simulink model "furuta_sim"  (R2020b)
settings: Solver=VariableStepAuto  StartTime=0.0  StopTime=10  MaxStep=1e-3  RelTol=1e-3
values from neighbouring files (symbols this model uses):
  A = A1    [furuta_script.m]    (also in practica2.m = [0 1; -2 -3])
  B = B1    [furuta_script.m]    (also in practica2.m = [10; 20])
  b1 = 1.00e-4    (= 0.0001)    [parameters.m]
  b2 = 2.80e-4    (= 0.00028)    [parameters.m]
  C = [1 0 0 0 0; 0 1 0 0 0]    [parameters.m]    (also in practica2.m = [1 0])
  CI = [-5*pi/180 -pi*5/180 0 0 0]    [furuta_script.m]
  g = 9.81    [parameters.m]
  J_hat_0 = J_hat_1+m2*L1^2    (= 0.0373463)    [parameters.m]
  J_hat_2 = J2+m2*l2^2    (= 0.0055028)    [parameters.m]
  K = acker(Pss.A, Pss.B, Pd)    [practica2_2.m]    (also in test_delete.m = Ka(1:3))
  Ki = -Ka(end)    [test_delete.m]
  Km = 0.090    (= 0.09)    [parameters.m]
  L = 0.005    [parameters.m]    (also in practica2_2.m = acker(Pss.A', Pss.c', Pdl)'; test_delete.m = acker(A',C',po)')
  L1 = 0.278    [parameters.m]
  l2 = 0.148    [parameters.m]
  m2 = 0.075    [parameters.m]
  n = length(A1)    [parameters.m]
  p = width(B1)    [parameters.m]    (also in test_delete.m = roots(conv([1 2*z*wn wn^2], [ 1 alpha*wn])))
  R = 7.80    (= 7.8)    [parameters.m]
undefined symbols (not defined in the file or in its folder): Kb, Nbar, Nbarb, Nbari
settings Model: Creator=jorgegonzales  LastModifiedBy=jorgegonzales

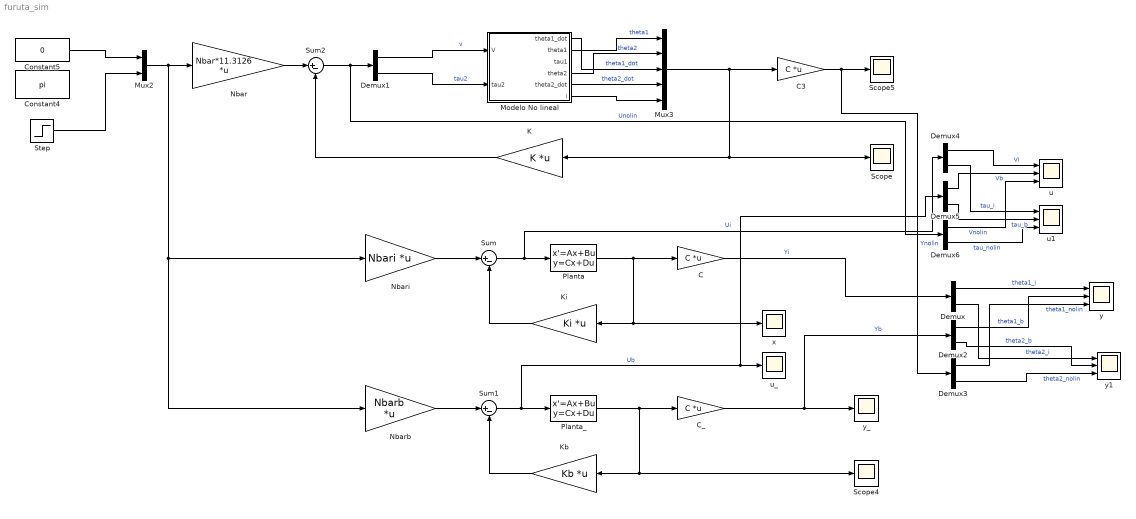
== system furuta_sim ==
  C : Gain  Gain=C  Multiplication=Matrix(K*u) (u vector)
  C3 : Gain  Gain=C  Multiplication=Matrix(K*u) (u vector)
  C_ : Gain  Gain=C  Multiplication=Matrix(K*u) (u vector)
  Constant4 : Constant  Value=pi
  Constant5 : Constant  Value=0
  Demux{,1..6} (7 alike) : Demux  Outputs=2
  K : Gain  Gain=K  Multiplication=Matrix(K*u) (u vector)
  Kb : Gain  Gain=Kb  Multiplication=Matrix(K*u) (u vector)
  Ki : Gain  Gain=Ki  Multiplication=Matrix(K*u) (u vector)
  Modelo No lineal : Subsystem
  Mux2 : Mux  Inputs=2
  Mux3 : Mux  Inputs=5
  Nbar : Gain  Gain=Nbar*11.3126  Multiplication=Matrix(K*u) (u vector)
  Nbarb : Gain  Gain=Nbarb  Multiplication=Matrix(K*u) (u vector)
  Nbari : Gain  Gain=Nbari  Multiplication=Matrix(K*u) (u vector)
  Planta : StateSpace  A=A  B=B  C=eye(n)  D=zeros(n,p)  InitialCondition=CI
  Planta_ : StateSpace  A=A  B=B  C=eye(n)  D=zeros(n,p)  InitialCondition=CI
  Scope : Scope
  Scope4 : Scope
  Scope5 : Scope
  Step : Step  Time=0.03  After=pi  SampleTime=0
  Sum : Sum  Inputs=|+-
  Sum1 : Sum  Inputs=|+-
  Sum2 : Sum  Inputs=|+-
  u : Scope  NumInputPorts=3
  u1 : Scope  NumInputPorts=3
  u_ : Scope
  x : Scope
  y : Scope  NumInputPorts=3
  y1 : Scope  NumInputPorts=3
  y_ : Scope
  wires:
  Ki/1 -> Sum/2
  Nbari/1 -> Sum/1
  Demux1/1 -> Modelo No lineal/1(V)  "v"
  Demux1/2 -> Modelo No lineal/2(tau2)  "tau2"
  C/1 -> Demux/1  "Yi"
  Planta/1 -> C/1, x/1, Ki/1
  Sum/1 -> Demux4/1, Planta/1  "Ui"
  Sum1/1 -> Demux5/1, u_/1, Planta_/1  "Ub"
  C_/1 -> Demux2/1, y_/1  "Yb"
  Planta_/1 -> Scope4/1, Kb/1, C_/1
  Nbarb/1 -> Sum1/1
  Kb/1 -> Sum1/2
  Constant5/1 -> Mux2/1
  Mux2/1 -> Nbarb/1, Nbari/1, Nbar/1
  Modelo No lineal/2(theta1) -> Mux3/1  "theta1"
  Modelo No lineal/4(theta2) -> Mux3/2  "theta2"
  Modelo No lineal/1(theta1_dot) -> Mux3/3  "theta1_dot"
  Modelo No lineal/5(theta2_dot) -> Mux3/4  "theta2_dot"
  Modelo No lineal/6(i) -> Mux3/5
  Mux3/1 -> C3/1, K/1, Scope/1
  C3/1 -> Demux3/1, Scope5/1  "Ynolin"
  Sum2/1 -> Demux6/1, Demux1/1  "Unolin"
  Nbar/1 -> Sum2/1
  K/1 -> Sum2/2
  Demux/1 -> y/1  "theta1_i"
  Demux2/1 -> y/2  "theta1_b"
  Demux3/1 -> y/3  "theta1_nolin"
  Demux/2 -> y1/1  "theta2_i"
  Demux2/2 -> y1/2  "theta2_b"
  Demux3/2 -> y1/3  "theta2_nolin"
  Demux4/1 -> u/1  "Vi"
  Demux4/2 -> u1/1  "tau_i"
  Demux5/1 -> u/2  "Vb"
  Demux5/2 -> u1/2  "tau_b"
  Demux6/1 -> u/3  "Vnolin"
  Demux6/2 -> u1/3  "tau_nolin"
  Step/1 -> Mux2/2

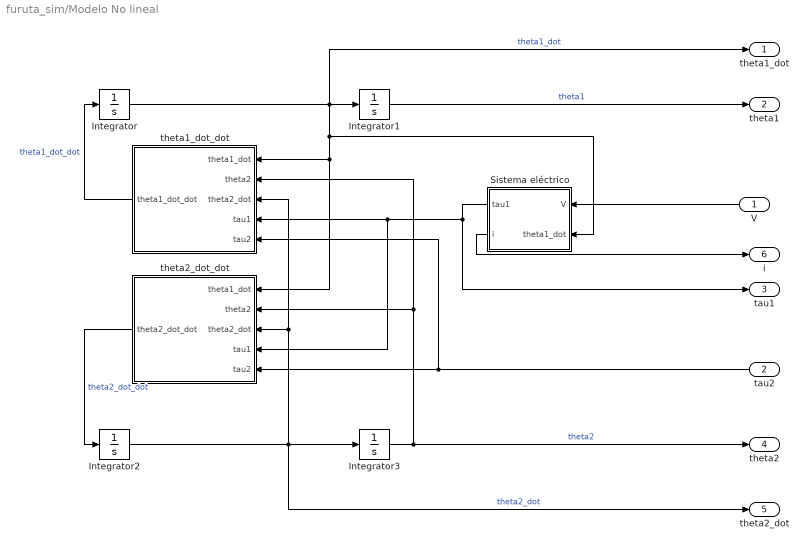
== system furuta_sim/Modelo No lineal ==
  V : Inport
  tau2 : Inport  Port=2
  Integrator : Integrator  InitialCondition=CI(3)
  Integrator1 : Integrator  InitialCondition=CI(1)
  Integrator2 : Integrator  InitialCondition=CI(4)
  Integrator3 : Integrator  InitialCondition=CI(2)
  Sistema eléctrico : Subsystem
  theta1_dot_dot : Subsystem
  theta2_dot_dot : Subsystem
  theta1_dot : Outport
  theta1 : Outport  Port=2
  tau1 : Outport  Port=3
  theta2 : Outport  Port=4
  theta2_dot : Outport  Port=5
  i : Outport  Port=6
  wires:
  Sistema eléctrico/1(tau1) -> tau1/1, theta2_dot_dot/4(tau1), theta1_dot_dot/4(tau1)
  theta1_dot_dot/1(theta1_dot_dot) -> Integrator/1  "theta1_dot_dot"
  V/1 -> Sistema eléctrico/1(V)
  Integrator3/1 -> theta2/1, theta2_dot_dot/2(theta2), theta1_dot_dot/2(theta2)  "theta2"
  tau2/1 -> theta1_dot_dot/5(tau2), theta2_dot_dot/5(tau2)
  theta2_dot_dot/1(theta2_dot_dot) -> Integrator2/1  "theta2_dot_dot"
  Integrator1/1 -> theta1/1  "theta1"
  Integrator2/1 -> theta2_dot/1, theta2_dot_dot/3(theta2_dot), theta1_dot_dot/3(theta2_dot), Integrator3/1  "theta2_dot"
  Integrator/1 -> theta1_dot/1, Sistema eléctrico/2(theta1_dot), theta1_dot_dot/1(theta1_dot), theta2_dot_dot/1(theta1_dot), Integrator1/1  "theta1_dot"
  Sistema eléctrico/2(i) -> i/1

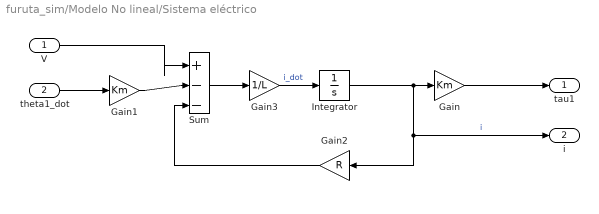
== system furuta_sim/Modelo No lineal/Sistema eléctrico ==
  V : Inport
  theta1_dot : Inport  Port=2
  Gain : Gain  Gain=Km
  Gain1 : Gain  Gain=Km
  Gain2 : Gain  Gain=R
  Gain3 : Gain  Gain=1/L
  Integrator : Integrator  InitialCondition=CI(5)
  Sum : Sum  Inputs=|+--
  tau1 : Outport
  i : Outport  Port=2
  wires:
  Integrator/1 -> i/1, Gain2/1, Gain/1  "i"
  Gain/1 -> tau1/1
  theta1_dot/1 -> Gain1/1
  Gain1/1 -> Sum/2
  V/1 -> Sum/1
  Gain2/1 -> Sum/3
  Gain3/1 -> Integrator/1  "i_dot"
  Sum/1 -> Gain3/1

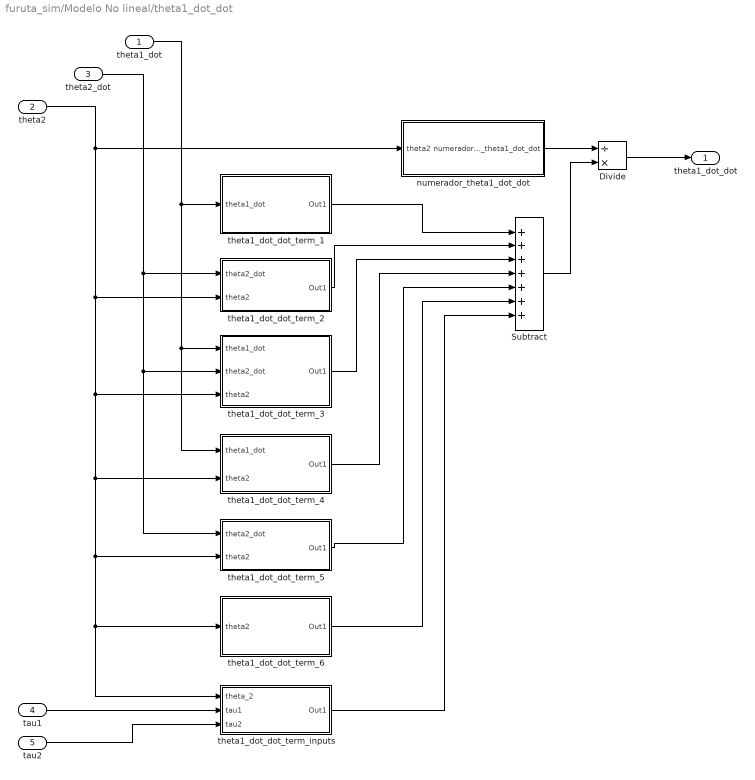
== system furuta_sim/Modelo No lineal/theta1_dot_dot ==
  theta1_dot : Inport
  theta2 : Inport  Port=2
  theta2_dot : Inport  Port=3
  tau1 : Inport  Port=4
  tau2 : Inport  Port=5
  Divide : Product  Inputs=/*
  Subtract : Sum  Inputs=+++++++
  numerador_theta1_dot_dot : Subsystem
  theta1_dot_dot_term_1 : Subsystem
  theta1_dot_dot_term_2 : Subsystem
  theta1_dot_dot_term_3 : Subsystem
  theta1_dot_dot_term_4 : Subsystem
  theta1_dot_dot_term_5 : Subsystem
  theta1_dot_dot_term_6 : Subsystem
  theta1_dot_dot_term_inputs : Subsystem
  theta1_dot_dot : Outport
  wires:
  theta1_dot_dot_term_4/1(Out1) -> Subtract/4
  theta1_dot/1 -> theta1_dot_dot_term_3/1(theta1_dot), theta1_dot_dot_term_4/1(theta1_dot), theta1_dot_dot_term_1/1(theta1_dot)
  theta1_dot_dot_term_3/1(Out1) -> Subtract/3
  theta1_dot_dot_term_5/1(Out1) -> Subtract/5
  theta1_dot_dot_term_2/1(Out1) -> Subtract/2
  theta1_dot_dot_term_1/1(Out1) -> Subtract/1
  theta2_dot/1 -> theta1_dot_dot_term_5/1(theta2_dot), theta1_dot_dot_term_3/2(theta2_dot), theta1_dot_dot_term_2/1(theta2_dot)
  theta2/1 -> numerador_theta1_dot_dot/1(theta2), theta1_dot_dot_term_4/2(theta2), theta1_dot_dot_term_6/1(theta2), theta1_dot_dot_term_inputs/1(theta_2), theta1_dot_dot_term_5/2(theta2), theta1_dot_dot_term_3/3(theta2), theta1_dot_dot_term_2/2(theta2)
  tau1/1 -> theta1_dot_dot_term_inputs/2(tau1)
  tau2/1 -> theta1_dot_dot_term_inputs/3(tau2)
  theta1_dot_dot_term_6/1(Out1) -> Subtract/6
  theta1_dot_dot_term_inputs/1(Out1) -> Subtract/7
  numerador_theta1_dot_dot/1(numerador_theta1_dot_dot) -> Divide/1
  Subtract/1 -> Divide/2
  Divide/1 -> theta1_dot_dot/1

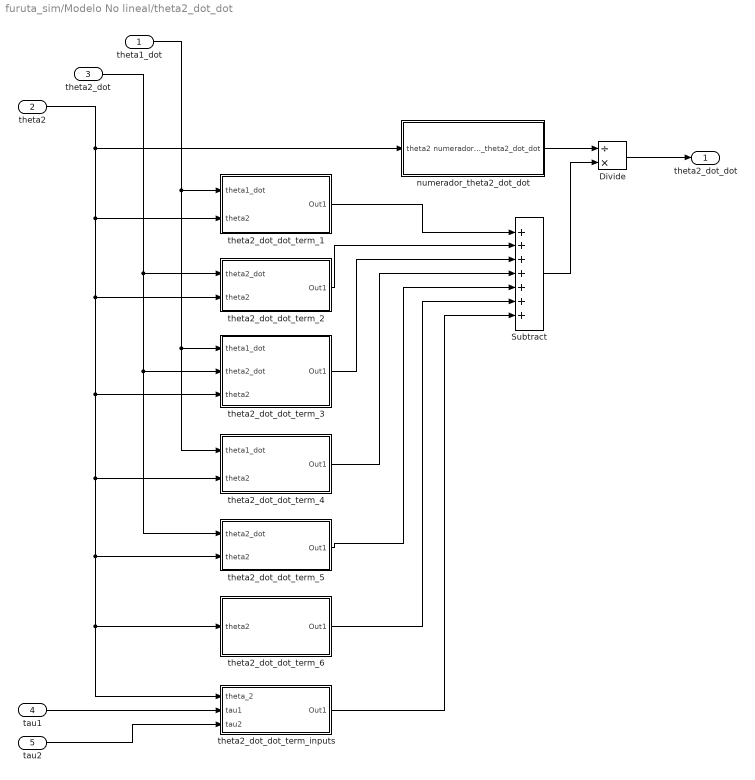
== system furuta_sim/Modelo No lineal/theta2_dot_dot ==
  theta1_dot : Inport
  theta2 : Inport  Port=2
  theta2_dot : Inport  Port=3
  tau1 : Inport  Port=4
  tau2 : Inport  Port=5
  Divide : Product  Inputs=/*
  Subtract : Sum  Inputs=+++++++
  numerador_theta2_dot_dot : Subsystem
  theta2_dot_dot_term_1 : Subsystem
  theta2_dot_dot_term_2 : Subsystem
  theta2_dot_dot_term_3 : Subsystem
  theta2_dot_dot_term_4 : Subsystem
  theta2_dot_dot_term_5 : Subsystem
  theta2_dot_dot_term_6 : Subsystem
  theta2_dot_dot_term_inputs : Subsystem
  theta2_dot_dot : Outport
  wires:
  Divide/1 -> theta2_dot_dot/1
  Subtract/1 -> Divide/2
  numerador_theta2_dot_dot/1(numerador_theta2_dot_dot) -> Divide/1
  theta2_dot_dot_term_inputs/1(Out1) -> Subtract/7
  theta2_dot_dot_term_6/1(Out1) -> Subtract/6
  tau2/1 -> theta2_dot_dot_term_inputs/3(tau2)
  tau1/1 -> theta2_dot_dot_term_inputs/2(tau1)
  theta2/1 -> theta2_dot_dot_term_1/2(theta2), theta2_dot_dot_term_2/2(theta2), theta2_dot_dot_term_3/3(theta2), theta2_dot_dot_term_5/2(theta2), theta2_dot_dot_term_inputs/1(theta_2), theta2_dot_dot_term_6/1(theta2), theta2_dot_dot_term_4/2(theta2), numerador_theta2_dot_dot/1(theta2)
  theta2_dot/1 -> theta2_dot_dot_term_2/1(theta2_dot), theta2_dot_dot_term_3/2(theta2_dot), theta2_dot_dot_term_5/1(theta2_dot)
  theta2_dot_dot_term_1/1(Out1) -> Subtract/1
  theta2_dot_dot_term_2/1(Out1) -> Subtract/2
  theta2_dot_dot_term_5/1(Out1) -> Subtract/5
  theta2_dot_dot_term_3/1(Out1) -> Subtract/3
  theta1_dot/1 -> theta2_dot_dot_term_4/1(theta1_dot), theta2_dot_dot_term_3/1(theta1_dot), theta2_dot_dot_term_1/1(theta1_dot)
  theta2_dot_dot_term_4/1(Out1) -> Subtract/4

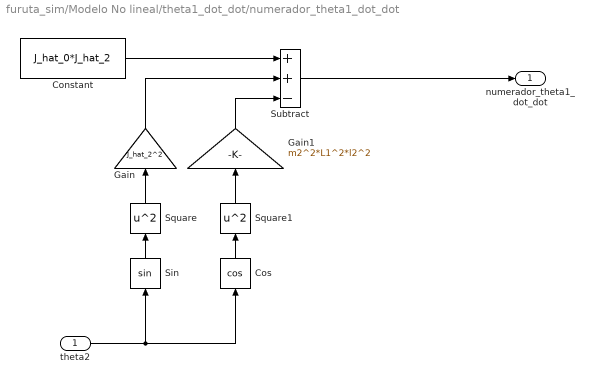
== system furuta_sim/Modelo No lineal/theta1_dot_dot/numerador_theta1_dot_dot ==
  theta2 : Inport
  Constant : Constant  Value=J_hat_0*J_hat_2
  Cos : Trigonometry  Operator=cos
  Gain : Gain  Gain=J_hat_2^2
  Gain1 : Gain  Gain=m2^2*L1^2*l2^2
  Sin : Trigonometry
  Square : Math  Operator=square  SaturateOnIntegerOverflow=on
  Square1 : Math  Operator=square  SaturateOnIntegerOverflow=on
  Subtract : Sum  Inputs=++-
  numerador_theta1_dot_dot : Outport
  wires:
  Subtract/1 -> numerador_theta1_dot_dot/1
  Gain1/1 -> Subtract/3
  Sin/1 -> Square/1
  Gain/1 -> Subtract/2
  Constant/1 -> Subtract/1
  theta2/1 -> Cos/1, Sin/1
  Cos/1 -> Square1/1
  Square/1 -> Gain/1
  Square1/1 -> Gain1/1

== system furuta_sim/Modelo No lineal/theta1_dot_dot/theta1_dot_dot_term_1 ==
  theta1_dot : Inport
  Gain2 : Gain  Gain=-1*J_hat_2*b1
  Out1 : Outport
  wires:
  theta1_dot/1 -> Gain2/1
  Gain2/1 -> Out1/1

== system furuta_sim/Modelo No lineal/theta1_dot_dot/theta1_dot_dot_term_2 ==
  theta2_dot : Inport
  theta2 : Inport  Port=2
  Cos1 : Trigonometry  Operator=cos
  Divide1 : Product  Inputs=**
  Gain3 : Gain  Gain=m2*L1*l2*b2
  Out1 : Outport
  wires:
  Gain3/1 -> Divide1/1
  theta2_dot/1 -> Divide1/2
  Cos1/1 -> Gain3/1
  theta2/1 -> Cos1/1
  Divide1/1 -> Out1/1

== system furuta_sim/Modelo No lineal/theta1_dot_dot/theta1_dot_dot_term_3 ==
  theta1_dot : Inport
  theta2_dot : Inport  Port=2
  theta2 : Inport  Port=3
  Divide2 : Product  Inputs=***
  Gain4 : Gain  Gain=2
  Gain5 : Gain  Gain=-1*J_hat_2^2
  Sin1 : Trigonometry
  Out1 : Outport
  wires:
  theta2_dot/1 -> Divide2/3
  Sin1/1 -> Gain5/1
  theta1_dot/1 -> Divide2/2
  Divide2/1 -> Out1/1
  theta2/1 -> Gain4/1
  Gain4/1 -> Sin1/1
  Gain5/1 -> Divide2/1

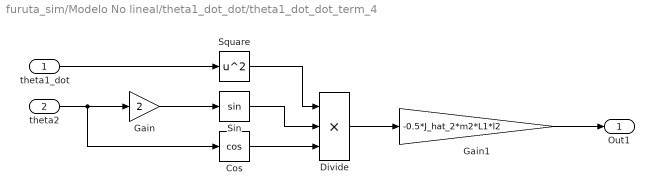
== system furuta_sim/Modelo No lineal/theta1_dot_dot/theta1_dot_dot_term_4 ==
  theta1_dot : Inport
  theta2 : Inport  Port=2
  Cos : Trigonometry  Operator=cos
  Divide : Product  Inputs=***
  Gain : Gain  Gain=2
  Gain1 : Gain  Gain=-0.5*J_hat_2*m2*L1*l2
  Sin : Trigonometry
  Square : Math  Operator=square  SaturateOnIntegerOverflow=on
  Out1 : Outport
  wires:
  Gain/1 -> Sin/1
  Divide/1 -> Gain1/1
  theta1_dot/1 -> Square/1
  Square/1 -> Divide/1
  Sin/1 -> Divide/2
  theta2/1 -> Cos/1, Gain/1
  Cos/1 -> Divide/3
  Gain1/1 -> Out1/1

== system furuta_sim/Modelo No lineal/theta1_dot_dot/theta1_dot_dot_term_5 ==
  theta2_dot : Inport
  theta2 : Inport  Port=2
  Divide : Product  Inputs=**
  Gain : Gain  Gain=J_hat_2*m2*L1*l2
  Sin : Trigonometry
  Square : Math  Operator=square  SaturateOnIntegerOverflow=on
  Out1 : Outport
  wires:
  theta2_dot/1 -> Square/1
  Square/1 -> Divide/2
  Sin/1 -> Divide/1
  Divide/1 -> Gain/1
  theta2/1 -> Sin/1
  Gain/1 -> Out1/1

== system furuta_sim/Modelo No lineal/theta1_dot_dot/theta1_dot_dot_term_6 ==
  theta2 : Inport
  Gain : Gain  Gain=2
  Gain1 : Gain  Gain=0.5*m2^2*l2^2*L1*g
  Sin : Trigonometry
  Out1 : Outport
  wires:
  theta2/1 -> Gain/1
  Gain1/1 -> Out1/1
  Gain/1 -> Sin/1
  Sin/1 -> Gain1/1

== system furuta_sim/Modelo No lineal/theta1_dot_dot/theta1_dot_dot_term_inputs ==
  theta_2 : Inport
  tau1 : Inport  Port=2
  tau2 : Inport  Port=3
  Cos : Trigonometry  Operator=cos
  Divide : Product  Inputs=**
  Gain : Gain  Gain=J_hat_2
  Gain1 : Gain  Gain=-1*m2*L1*l2
  Sum : Sum  Inputs=|++
  Out1 : Outport
  wires:
  theta_2/1 -> Cos/1
  Sum/1 -> Out1/1
  Gain/1 -> Sum/1
  Cos/1 -> Divide/2
  tau1/1 -> Gain/1
  tau2/1 -> Divide/1
  Gain1/1 -> Sum/2
  Divide/1 -> Gain1/1

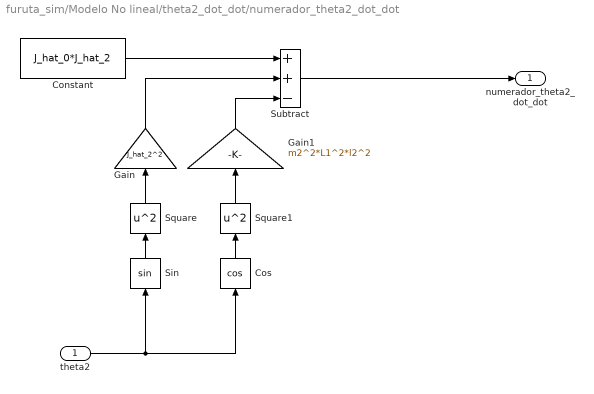
== system furuta_sim/Modelo No lineal/theta2_dot_dot/numerador_theta2_dot_dot ==
  theta2 : Inport
  Constant : Constant  Value=J_hat_0*J_hat_2
  Cos : Trigonometry  Operator=cos
  Gain : Gain  Gain=J_hat_2^2
  Gain1 : Gain  Gain=m2^2*L1^2*l2^2
  Sin : Trigonometry
  Square : Math  Operator=square  SaturateOnIntegerOverflow=on
  Square1 : Math  Operator=square  SaturateOnIntegerOverflow=on
  Subtract : Sum  Inputs=++-
  numerador_theta2_dot_dot : Outport
  wires:
  Square1/1 -> Gain1/1
  Square/1 -> Gain/1
  Cos/1 -> Square1/1
  theta2/1 -> Cos/1, Sin/1
  Constant/1 -> Subtract/1
  Gain/1 -> Subtract/2
  Sin/1 -> Square/1
  Gain1/1 -> Subtract/3
  Subtract/1 -> numerador_theta2_dot_dot/1

== system furuta_sim/Modelo No lineal/theta2_dot_dot/theta2_dot_dot_term_1 ==
  theta1_dot : Inport
  theta2 : Inport  Port=2
  Cos : Trigonometry  Operator=cos
  Divide : Product  Inputs=**
  Gain2 : Gain  Gain=m2*L1*l2*b1
  Out1 : Outport
  wires:
  Gain2/1 -> Out1/1
  theta2/1 -> Cos/1
  Cos/1 -> Divide/2
  theta1_dot/1 -> Divide/1
  Divide/1 -> Gain2/1

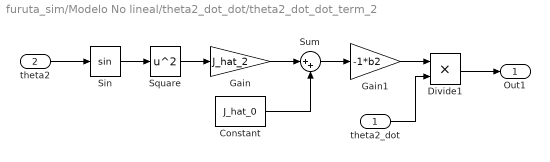
== system furuta_sim/Modelo No lineal/theta2_dot_dot/theta2_dot_dot_term_2 ==
  theta2_dot : Inport
  theta2 : Inport  Port=2
  Constant : Constant  Value=J_hat_0
  Divide1 : Product  Inputs=**
  Gain : Gain  Gain=J_hat_2
  Gain1 : Gain  Gain=-1*b2
  Sin : Trigonometry
  Square : Math  Operator=square  SaturateOnIntegerOverflow=on
  Sum : Sum  Inputs=|++
  Out1 : Outport
  wires:
  Divide1/1 -> Out1/1
  theta2/1 -> Sin/1
  Sin/1 -> Square/1
  Square/1 -> Gain/1
  Gain/1 -> Sum/1
  Constant/1 -> Sum/2
  Sum/1 -> Gain1/1
  Gain1/1 -> Divide1/1
  theta2_dot/1 -> Divide1/2

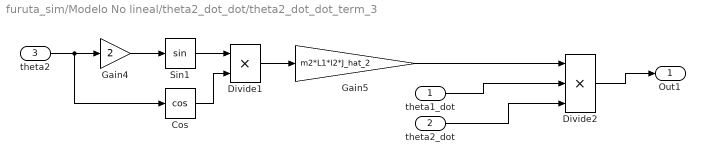
== system furuta_sim/Modelo No lineal/theta2_dot_dot/theta2_dot_dot_term_3 ==
  theta1_dot : Inport
  theta2_dot : Inport  Port=2
  theta2 : Inport  Port=3
  Cos : Trigonometry  Operator=cos
  Divide1 : Product  Inputs=**
  Divide2 : Product  Inputs=***
  Gain4 : Gain  Gain=2
  Gain5 : Gain  Gain=m2*L1*l2*J_hat_2
  Sin1 : Trigonometry
  Out1 : Outport
  wires:
  Gain5/1 -> Divide2/1
  Gain4/1 -> Sin1/1
  theta2/1 -> Cos/1, Gain4/1
  Divide2/1 -> Out1/1
  theta1_dot/1 -> Divide2/2
  theta2_dot/1 -> Divide2/3
  Sin1/1 -> Divide1/1
  Cos/1 -> Divide1/2
  Divide1/1 -> Gain5/1

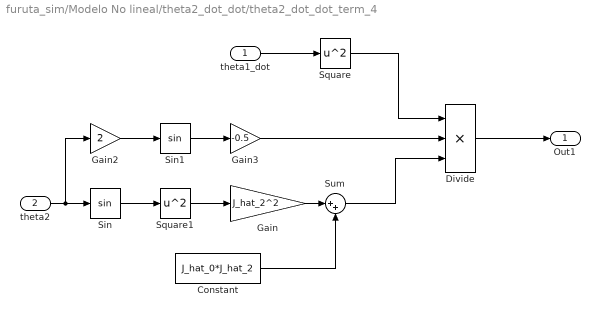
== system furuta_sim/Modelo No lineal/theta2_dot_dot/theta2_dot_dot_term_4 ==
  theta1_dot : Inport
  theta2 : Inport  Port=2
  Constant : Constant  Value=J_hat_0*J_hat_2
  Divide : Product  Inputs=***
  Gain : Gain  Gain=J_hat_2^2
  Gain2 : Gain  Gain=2
  Gain3 : Gain  Gain=-0.5
  Sin : Trigonometry
  Sin1 : Trigonometry
  Square : Math  Operator=square  SaturateOnIntegerOverflow=on
  Square1 : Math  Operator=square  SaturateOnIntegerOverflow=on
  Sum : Sum  Inputs=|++
  Out1 : Outport
  wires:
  Divide/1 -> Out1/1
  Square/1 -> Divide/1
  theta1_dot/1 -> Square/1
  theta2/1 -> Gain2/1, Sin/1
  Sin/1 -> Square1/1
  Square1/1 -> Gain/1
  Gain/1 -> Sum/1
  Constant/1 -> Sum/2
  Gain2/1 -> Sin1/1
  Sin1/1 -> Gain3/1
  Gain3/1 -> Divide/2
  Sum/1 -> Divide/3

== system furuta_sim/Modelo No lineal/theta2_dot_dot/theta2_dot_dot_term_5 ==
  theta2_dot : Inport
  theta2 : Inport  Port=2
  Divide : Product  Inputs=**
  Gain : Gain  Gain=-0.5*m2^2*L1^2*l2^2
  Gain1 : Gain  Gain=2
  Sin : Trigonometry
  Square : Math  Operator=square  SaturateOnIntegerOverflow=on
  Out1 : Outport
  wires:
  Gain/1 -> Out1/1
  Divide/1 -> Gain/1
  Sin/1 -> Divide/1
  Square/1 -> Divide/2
  theta2_dot/1 -> Square/1
  theta2/1 -> Gain1/1
  Gain1/1 -> Sin/1

== system furuta_sim/Modelo No lineal/theta2_dot_dot/theta2_dot_dot_term_6 ==
  theta2 : Inport
  Constant : Constant  Value=J_hat_0
  Divide : Product  Inputs=**
  Gain : Gain  Gain=J_hat_2
  Gain1 : Gain  Gain=-1*m2*l2*g
  Sin : Trigonometry
  Square : Math  Operator=square  SaturateOnIntegerOverflow=on
  Sum : Sum  Inputs=|++
  Out1 : Outport
  wires:
  Gain1/1 -> Out1/1
  theta2/1 -> Sin/1
  Sin/1 -> Divide/1, Square/1
  Square/1 -> Gain/1
  Gain/1 -> Sum/1
  Constant/1 -> Sum/2
  Sum/1 -> Divide/2
  Divide/1 -> Gain1/1

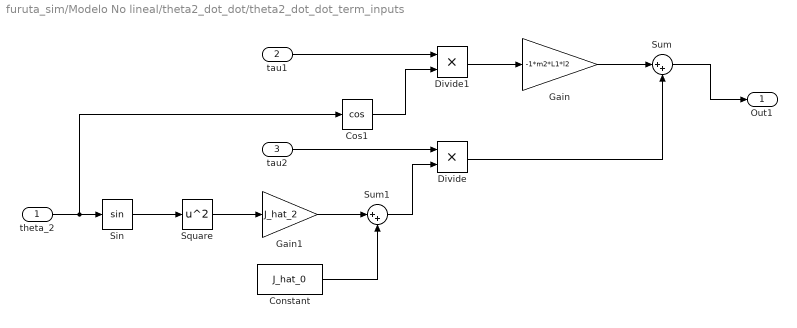
== system furuta_sim/Modelo No lineal/theta2_dot_dot/theta2_dot_dot_term_inputs ==
  theta_2 : Inport
  tau1 : Inport  Port=2
  tau2 : Inport  Port=3
  Constant : Constant  Value=J_hat_0
  Cos1 : Trigonometry  Operator=cos
  Divide : Product  Inputs=**
  Divide1 : Product  Inputs=**
  Gain : Gain  Gain=-1*m2*L1*l2
  Gain1 : Gain  Gain=J_hat_2
  Sin : Trigonometry
  Square : Math  Operator=square  SaturateOnIntegerOverflow=on
  Sum : Sum  Inputs=|++
  Sum1 : Sum  Inputs=|++
  Out1 : Outport
  wires:
  Divide/1 -> Sum/2
  tau2/1 -> Divide/1
  Sum/1 -> Out1/1
  tau1/1 -> Divide1/1
  Cos1/1 -> Divide1/2
  Gain/1 -> Sum/1
  Divide1/1 -> Gain/1
  theta_2/1 -> Cos1/1, Sin/1
  Sin/1 -> Square/1
  Square/1 -> Gain1/1
  Gain1/1 -> Sum1/1
  Constant/1 -> Sum1/2
  Sum1/1 -> Divide/2
